simulink model "BatteryModelDifferentialEquations"  (R2023b)
settings: Solver=VariableStepAuto  StartTime=0.0  StopTime=41000  RelTol=1e-3
values from neighbouring files (symbols this model uses):
  C1 = 12.6138    [DPBatteryDynamics.m]    (also in DPBatteryModuleDynamics.m = 174.354594213; MPCControllerForModuleSim.m = 174.354594213; StateSpaceScript.m; TubeBasedMPCControllerForModuleSim.m = 174.354594213)
  Cc = 62.7    [DPBatteryDynamics.m]    (also in DPBatteryModuleDynamics.m = 2059.88437317; MPCControllerForModuleSim.m = 2059.88437317; StateSpaceScript.m; TubeBasedMPCControllerForModuleSim.m = 2059.88437317)
  Cn = 78    [DPBatteryDynamics.m]    (also in DPBatteryModuleDynamics.m = 156; MPCControllerForModuleSim.m = 156; StateSpaceScript.m; TubeBasedMPCControllerForModuleSim.m = 156)
  Cs = 4.5    [DPBatteryDynamics.m]    (also in DPBatteryModuleDynamics.m = 31.8813725212; MPCControllerForModuleSim.m = 31.8813725212; StateSpaceScript.m; TubeBasedMPCControllerForModuleSim.m = 31.8813725212)
  R0 = 0.0099131    [DPBatteryDynamics.m]    (also in DPBatteryModuleDynamics.m = 0.000127631043389; FMINCONControllerForCellSim.m = 0.00292724690916; MPCControllerForModuleSim.m = 0.000127631043389; StateSpaceScript.m)
  R1 = 3e-4    (= 0.0003)    [DPBatteryDynamics.m]    (also in DPBatteryModuleDynamics.m = 0.00360795873337; MPCControllerForModuleSim.m = 0.00360795873337; StateSpaceScript.m; TubeBasedMPCControllerForModuleSim.m = 0.00360795873337)
  Rc = 1.94    [DPBatteryDynamics.m]    (also in DPBatteryModuleDynamics.m = 14.480191951; MPCControllerForModuleSim.m = 14.480191951; StateSpaceScript.m; TubeBasedMPCControllerForModuleSim.m = 14.480191951)
  Ru = 15    [DPBatteryDynamics.m]    (also in DPBatteryModuleDynamics.m = 8.86466905699; MPCControllerForModuleSim.m = 8.86466905699; StateSpaceScript.m; TubeBasedMPCControllerForModuleSim.m = 8.86466905699)
  Tf = 20    [DPBatteryDynamics.m]    (also in DPBatteryModuleDynamics.m; MPCControllerForModuleSim.m; RHC_test.m; StateSpaceScript.m)
libraries: simulink x1
settings Model: Creator=adamb  LastModifiedBy=Adam

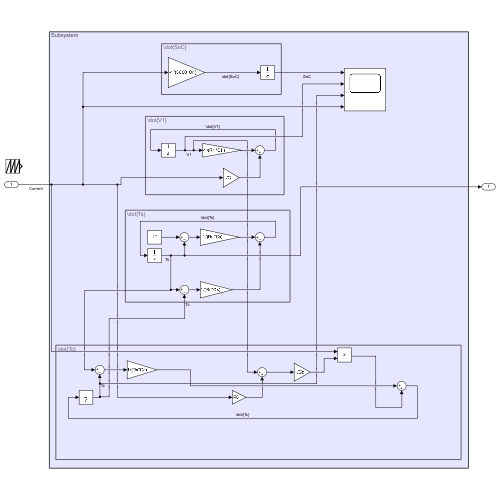
[thumbnail: Simulink's stored preview of the top-level diagram]
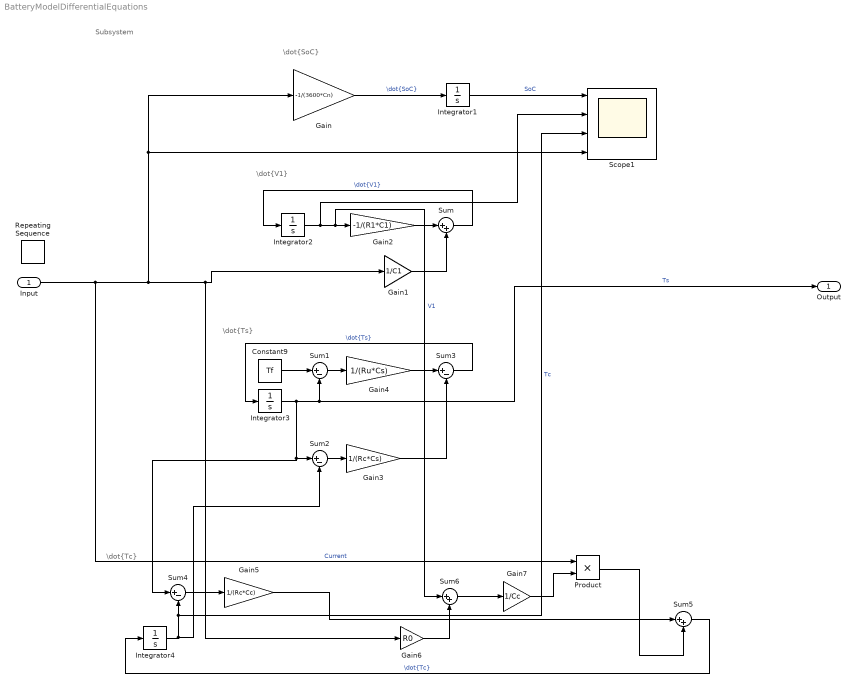
== system BatteryModelDifferentialEquations ==
  note: Subsystem
  note: \dot{V1}
  note: \dot{SoC}
  note: \dot{Ts}
  note: \dot{Tc}
  Input : Inport
  Constant9 : Constant  Value=Tf
  Gain : Gain  Gain=-1/(3600*Cn)
  Gain1 : Gain  Gain=1/C1
  Gain2 : Gain  Gain=-1/(R1*C1)
  Gain3 : Gain  Gain=1/(Rc*Cs)
  Gain4 : Gain  Gain=1/(Ru*Cs)
  Gain5 : Gain  Gain=1/(Rc*Cc)
  Gain6 : Gain  Gain=R0
  Gain7 : Gain  Gain=1/Cc
  Integrator1 : Integrator  InitialCondition=1
  Integrator2 : Integrator
  Integrator3 : Integrator  InitialCondition=Tf
  Integrator4 : Integrator  InitialCondition=Tf
  Product : Product
  Repeating Sequence : simulink/Sources/Repeating Sequence  rep_seq_t=sim_time  rep_seq_y=input_current
  Scope1 : Scope  NumInputPorts=4
  Sum : Sum  Inputs=|++
  Sum{1..4} (4 alike) : Sum  Inputs=|+-
  Sum5 : Sum  Inputs=|++
  Sum6 : Sum  Inputs=|++
  Output : Outport  PortDimensions=2
  wires:
  Input/1 -> Gain1/1, Gain6/1, Scope1/4, Gain/1, Product/1  "Current"
  Sum3/1 -> Integrator3/1  "\\dot{Ts}"
  Sum2/1 -> Gain3/1
  Sum1/1 -> Gain4/1
  Product/1 -> Sum5/2
  Gain/1 -> Integrator1/1  "\\dot{SoC}"
  Gain2/1 -> Sum/1
  Gain7/1 -> Product/2
  Gain5/1 -> Sum5/1
  Constant9/1 -> Sum1/1
  Integrator2/1 -> Sum6/1, Gain2/1, Scope1/2  "V1"
  Gain6/1 -> Sum6/2
  Gain3/1 -> Sum3/2
  Sum4/1 -> Gain5/1
  Integrator3/1 -> Sum4/1, Sum2/1, Output/1, Sum1/2  "Ts"
  Sum5/1 -> Integrator4/1  "\\dot{Tc}"
  Integrator1/1 -> Scope1/1  "SoC"
  Integrator4/1 -> Sum2/2, Scope1/3, Sum4/2  "Tc"
  Sum/1 -> Integrator2/1  "\\dot{V1}"
  Sum6/1 -> Gain7/1
  Gain4/1 -> Sum3/1
  Gain1/1 -> Sum/2
